simulink library "Index2DbTable"  (R2022b)
settings: Solver=VariableStepAuto  StartTime=0.0  StopTime=10.0  RelTol=1e-3
undefined symbols (not defined in the file or in its folder): MaskRows, MaskVolumeTable
libraries: Index2DbTableBtc x1
settings Model: Creator=kl13806  LastModifiedBy=kl13806
settings SolverCC: AlgebraicLoopSolver=TrustRegion
settings DebuggingCC: UnconnectedInputMsg=warning  UnconnectedOutputMsg=warning  UnconnectedLineMsg=warning  SFMachineParentedDataDiag=warning  ArithmeticOperatorsInVariantConditions=warning
settings ModelReferenceCC: EnableRefExpFcnMdlSchedulingChecks=on
settings SFSimCC: CustomCodeUndefinedFunction=UseInterfaceOnly
settings RTWCC: DLArmComputeVersion=19.05

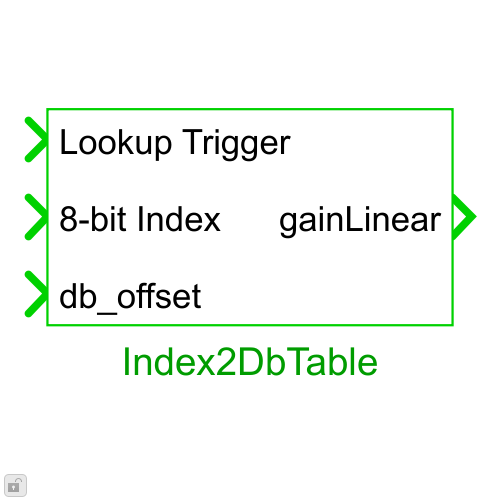
[thumbnail: Simulink's stored preview of the top-level diagram]
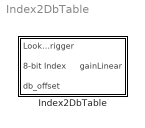
== system Index2DbTable ==
  Index2DbTable : Subsystem  mask(Bose Index-to-dB Table){MaskRows=MaskRows, MaskValue=MaskVolumeTable, BankNumber=[]}
      mask prompts: MaskRows "Maximum Table Points:"; MaskValue "Default Table:"; BankNumber "Bank number:"
      mask help: This block contains overlay tuning data for an index-to-dB lookup table. Provide the maximum number of points in the table as a build-time variable. The TuneVar is variable size, but must define at least two points (i.e. two rows, or four values).
      mask init:
      | blkh = gcbh;
      | % Copy discrete mask parameters into a classdef object
      | InnerLinkConfig = Index2DbTableConfig;
      | InnerLinkConfig.MaximumTablePoints = MaskRows;
      | InnerLinkConfig.DefaultTable = MaskValue;
      | InnerLinkConfig.BankNumber = BankNumber;
      mask Help:
      | This block contains overlay tuning data which defines an index-to-dB lookup table.
      | Each row of the tuning data contains an index and a dB value.
      | 
      | Tuning data
      | ---------------
      |    tune index: normalized value between 0 and 1
      |    tune value: dB value such as 0 (aka linear "1") or -100 (aka "very quiet")
      | 
      | Inports
      | ----------
      |    trigger: function call trigger that invokes the lookup from inport index to output dB
      |    index: an 8-bit integer index between [0:255] corresponding to the tuning index range [0:1]
      | 
      | Outport
      | -----------
      |    The resulting dB value looked up in the tuned table by using the inbound index
      mask DialogControl SelectPackage Prompt: Select
      mask DialogControl SelectPackage Callback: TuneVarMask.CB_SelectPackage(gcbh);

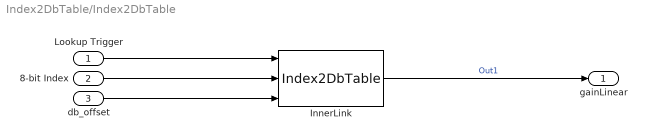
== system Index2DbTable/Index2DbTable ==
  Lookup Trigger : Inport
  8-bit Index : Inport  Port=2
  db_offset : Inport  Port=3
  InnerLink : Index2DbTableBtc/Index2DbTable  Config=InnerLinkConfig
      settings: SourceProductName=Bose Blocklib
  gainLinear : Outport
  wires:
  InnerLink/1 -> gainLinear/1  "Out1"
  Lookup Trigger/1 -> InnerLink/1
  8-bit Index/1 -> InnerLink/2
  db_offset/1 -> InnerLink/3
